simulink model "myo_model_w_ctrl"  (R2020b)
settings: Solver=VariableStepAuto  StartTime=0.0  StopTime=4  RelTol=1e-3
values from neighbouring files (symbols this model uses):
  beta_force = 3    [project_myo.m]
  beta_force_int = 4    [project_myo.m]
  beta_pos = 4    [project_myo.m]
  d = 0.01    [project_myo.m]
  j = 0.068    [project_myo.m]
  Kd = 2    [project_myo.m]
  Kp = 140    [project_myo.m]
libraries: cstblocks x3
settings Model: Creator=simon  LastModifiedBy=simon

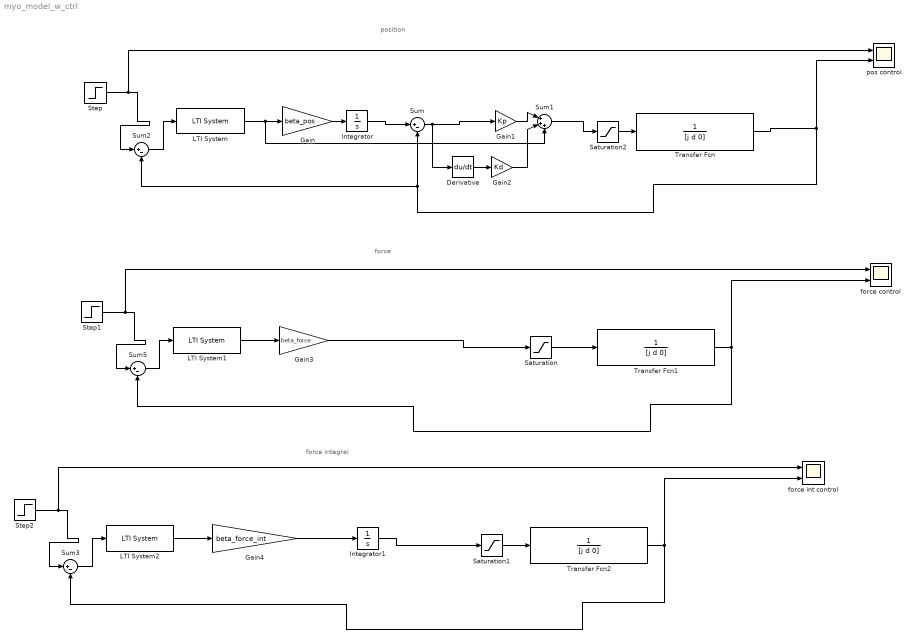
== system myo_model_w_ctrl ==
  note: position
  note: force
  note: force integral
  Derivative : Derivative
  Gain : Gain  Gain=beta_pos
  Gain1 : Gain  Gain=Kp
  Gain2 : Gain  Gain=Kd
  Gain3 : Gain  Gain=beta_force
  Gain4 : Gain  Gain=beta_force_int
  Integrator : Integrator
  Integrator1 : Integrator
  LTI System : cstblocks/LTI System  sys=bestCtrlModel  IC=[]
  LTI System1 : cstblocks/LTI System  sys=bestCtrlModel  IC=[]
  LTI System2 : cstblocks/LTI System  sys=bestCtrlModel  IC=[]
  Saturation : Saturate  UpperLimit=6  LowerLimit=-6
  Saturation1 : Saturate  UpperLimit=6  LowerLimit=-6
  Saturation2 : Saturate  UpperLimit=6  LowerLimit=-6
  Step : Step  Time=0  SampleTime=0
  Step1 : Step  Time=0  SampleTime=0
  Step2 : Step  Time=0  SampleTime=0
  Sum{,2..3,5} (4 alike) : Sum  Inputs=|+-
  Sum1 : Sum  Inputs=|+++
  Transfer Fcn : TransferFcn  Denominator=[j d 0]
  Transfer Fcn1 : TransferFcn  Denominator=[j d 0]
  Transfer Fcn2 : TransferFcn  Denominator=[j d 0]
  force control : Scope  NumInputPorts=2
  force int control : Scope  NumInputPorts=2
  pos control : Scope  NumInputPorts=2
  wires:
  Gain/1 -> Integrator/1
  Derivative/1 -> Gain2/1
  Sum/1 -> Derivative/1, Gain1/1
  Gain1/1 -> Sum1/1
  Gain2/1 -> Sum1/2
  Sum1/1 -> Saturation2/1
  Transfer Fcn/1 -> pos control/2, Sum2/2, Sum/2
  Integrator/1 -> Sum/1
  LTI System/1 -> Sum1/3, Gain/1
  Step/1 -> pos control/1, Sum2/1
  Sum2/1 -> LTI System/1
  Sum5/1 -> LTI System1/1
  Transfer Fcn1/1 -> Sum5/2, force control/2
  Step1/1 -> force control/1, Sum5/1
  Gain3/1 -> Saturation/1
  LTI System1/1 -> Gain3/1
  LTI System2/1 -> Gain4/1
  Step2/1 -> force int control/1, Sum3/1
  Transfer Fcn2/1 -> Sum3/2, force int control/2
  Gain4/1 -> Integrator1/1
  Sum3/1 -> LTI System2/1
  Integrator1/1 -> Saturation1/1
  Saturation/1 -> Transfer Fcn1/1
  Saturation1/1 -> Transfer Fcn2/1
  Saturation2/1 -> Transfer Fcn/1
